simulink model "gm_uz_pmsm_model_9ph"  (R2021a)
settings: Solver=FixedStepAuto  StartTime=0.0  StopTime=.5  RelTol=1e-3
PreLoadFcn:
  | uz_pmsm_model_init_parameter
undefined symbols (not defined in the file or in its folder): friction_coefficient, inertia, k_i_d, k_p_d, k_p_q, L_d, L_o1, L_o2, L_q, L_x1, L_x2, L_y1, L_y2, L_zero, polepair, psi_pm, R_1, static_friction_torque
libraries: hdlmdlgenlib x220, hdlsllib x18, simulink x3, pid_lib x2
(part 1 of 4)
settings Model: Creator=ts  LastModifiedBy=valen
settings SolverCC: AlgebraicLoopSolver=TrustRegion  AutoInsertRateTranBlk=on
settings DataIOCC: LimitDataPoints=on  SaveOutput=off  SaveTime=off
settings OptimizationCC: BlockReduction=off  ConditionallyExecuteInputs=off  DefaultParameterBehavior=Inlined  LifeSpan=inf
settings DebuggingCC: AlgebraicLoopMsg=error  ArtificialAlgebraicLoopMsg=none  InheritedTsInSrcMsg=none  SingleTaskRateTransMsg=error  AllowSymbolicDim=off  StrictBusMsg=ErrorOnBusTreatedAsVector  SFUnexpectedBacktrackingDiag=warning  SFNoUnconditionalDefaultTransitionDiag=warning  SFExecutionAtInitializationDiag=none  SFMachineParentedDataDiag=warning  ArithmeticOperatorsInVariantConditions=warning
settings HardwareCC: ProdBitPerPointer=32  ProdBitPerSizeT=32  ProdBitPerPtrDiffT=32  ProdLargestAtomicFloat=None  ProdIntDivRoundTo=Undefined  ProdEndianess=Unspecified  ProdWordSize=32  ProdHWDeviceType=ASIC/FPGA->ASIC/FPGA  ProdEqTarget=off
settings SFSimCC: SimUseLocalCustomCode=off  CustomCodeUndefinedFunction=UseInterfaceOnly
settings RTWCC: RTWUseLocalCustomCode=off
settings CodeAppCC: StateflowObjectComments=on
settings GRTTargetCC: TargetLangStandard=C89/C90 (ANSI)
settings ConfigComp: CovScope=ReferencedModels  CovMetricSettings=dw  CovSaveCumulativeToWorkspaceVar=on  CovSaveSingleToWorkspaceVar=on  CovExternalEMLEnable=off  CovSFcnEnable=off

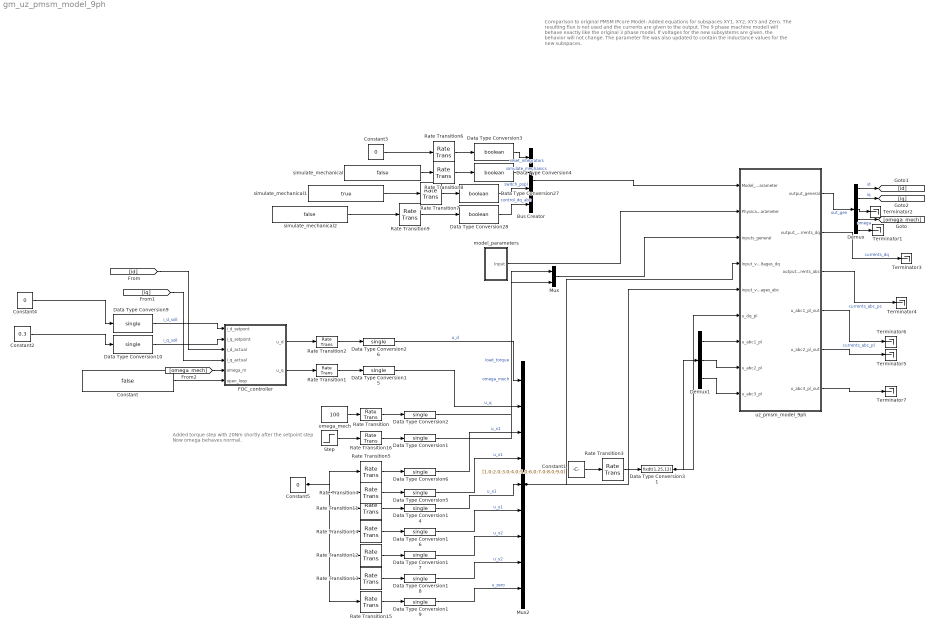
== system gm_uz_pmsm_model_9ph ==
  note: Comparison to original PMSM IPcore Model:
      | Added equations for subspaces XY1, XY2, XY3 and Zero. The resulting flux is not used and the currents are given to the output.
      | The 9 phase machine modell will behave exactly like the original 3 phase model. If voltages for the new subsystems are given, the behavior will not change.
      | The parameter file was also updated to contain the inductance values for the new subspaces.
  note: Added torque step with 20Nm shortly after the setpoint step
      | Now omega behaves normal.
  Bus Creator : BusCreator  Inputs=4
  Constant : Constant  Value=false
  Constant1 : Constant  Value=[1.0;2.0;3.0;4.0;5.0;6.0;7.0;8.0;9.0]
  Constant2 : Constant  Value=0.3
  Constant3 : Constant  Value=0
  Constant4 : Constant  Value=0
  Constant5 : Constant  Value=0
  Data Type Conversion{1..2,5..6,14..19,26} (11 alike) : DataTypeConversion  OutDataTypeStr=single  RndMeth=Nearest
  Data Type Conversion10 : DataTypeConversion  OutDataTypeStr=single
  Data Type Conversion{3..4,27..28} (4 alike) : DataTypeConversion  OutDataTypeStr=boolean
  Data Type Conversion31 : DataTypeConversion  OutDataTypeStr=fixdt(1,25,12)  RndMeth=Nearest
  Data Type Conversion9 : DataTypeConversion  OutDataTypeStr=single
  Demux : Demux  Outputs=5
  Demux1 : Demux  Outputs=3
  FOC_controller : Subsystem
  Mux : Mux  Inputs=2
  Mux2 : Mux  Inputs=9
  Rate Transition{,1..9,11..16} (16 alike) : RateTransition  OutPortSampleTime=ts
  Step : Step  Time=0.25  After=20  SampleTime=0
  Terminator{1..7} (7 alike) : Terminator
  model_parameters : Subsystem
  omega_mech : Constant  Value=100
  simulate_mechanical : Constant  Value=false
  simulate_mechanical1 : Constant  Value=true
  simulate_mechanical2 : Constant  Value=false
  uz_pmsm_model_9ph : Subsystem  TreatAsAtomicUnit=on
  wires:
  uz_pmsm_model_9ph/5(u_abc2_pl_out) -> Terminator5/1
  uz_pmsm_model_9ph/6(u_abc3_pl_out) -> Terminator7/1
  Demux1/3 -> uz_pmsm_model_9ph/9(u_abc3_pl)
  Demux1/2 -> uz_pmsm_model_9ph/8(u_abc2_pl)
  Demux1/1 -> uz_pmsm_model_9ph/7(u_abc1_pl)
  Rate Transition9/1 -> Data Type Conversion28/1
  Rate Transition7/1 -> Data Type Conversion27/1
  Data Type Conversion5/1 -> Mux2/4  "u_x1"
  Data Type Conversion6/1 -> Mux2/3  "u_x1"
  Rate Transition5/1 -> Data Type Conversion6/1
  Rate Transition4/1 -> Data Type Conversion5/1
  Data Type Conversion15/1 -> Mux2/2  "u_q"
  Data Type Conversion26/1 -> Mux2/1  "u_d"
  Demux/3 -> Terminator2/1
  Demux/5 -> Terminator1/1
  Constant2/1 -> Data Type Conversion10/1
  [id] -> FOC_controller/3(i_d_actual)
  [iq] -> FOC_controller/4(i_q_actual)
  Demux/2 -> [iq]  "iq"
  Demux/1 -> [id]  "id"
  Demux/4 -> [omega_mech]  "omega"
  [omega_mech] -> FOC_controller/5(omega_m)
  simulate_mechanical2/1 -> Rate Transition9/1
  simulate_mechanical1/1 -> Rate Transition7/1
  uz_pmsm_model_9ph/4(u_abc1_pl_out) -> Terminator6/1  "currents_abc_pl"
  Data Type Conversion31/1 -> uz_pmsm_model_9ph/6(u_dq_pl), Demux1/1
  Rate Transition3/1 -> Data Type Conversion31/1
  Constant1/1 -> Rate Transition3/1
  Data Type Conversion1/1 -> Mux/2  "load_torque"
  Data Type Conversion2/1 -> Mux/1  "omega_mech"
  Mux/1 -> uz_pmsm_model_9ph/3(inputs_general)
  Mux2/1 -> uz_pmsm_model_9ph/4(input_voltages_dq), uz_pmsm_model_9ph/5(input_voltages_abc)
  uz_pmsm_model_9ph/3(output_currents_abc) -> Terminator4/1  "currents_abc_ps"
  uz_pmsm_model_9ph/2(output_currents_dq) -> Terminator3/1  "currents_dq"
  Bus Creator/1 -> uz_pmsm_model_9ph/1(Model_Parameter)
  Data Type Conversion28/1 -> Bus Creator/4  "control_dq_abc"
  Data Type Conversion27/1 -> Bus Creator/3  "switch_pspl"
  Data Type Conversion3/1 -> Bus Creator/1  "reset_integrators"
  Data Type Conversion4/1 -> Bus Creator/2  "simulate_mechanics"
  model_parameters/1(Input) -> uz_pmsm_model_9ph/2(Physical_Parameter)
  Constant5/1 -> Rate Transition5/1, Rate Transition4/1, Rate Transition11/1, Rate Transition14/1, Rate Transition12/1, Rate Transition13/1, Rate Transition15/1
  Rate Transition15/1 -> Data Type Conversion19/1
  Data Type Conversion19/1 -> Mux2/9  "u_zero"
  Data Type Conversion18/1 -> Mux2/8  "u_y2"
  Data Type Conversion17/1 -> Mux2/7  "u_x2"
  Data Type Conversion16/1 -> Mux2/6  "u_y1"
  Rate Transition14/1 -> Data Type Conversion16/1
  Rate Transition12/1 -> Data Type Conversion17/1
  Rate Transition13/1 -> Data Type Conversion18/1
  Data Type Conversion14/1 -> Mux2/5  "u_x1"
  Rate Transition11/1 -> Data Type Conversion14/1
  Constant/1 -> FOC_controller/6(open_loop)
  omega_mech/1 -> Rate Transition/1
  FOC_controller/2(u_q) -> Rate Transition1/1
  FOC_controller/1(u_d) -> Rate Transition2/1
  Data Type Conversion10/1 -> FOC_controller/2(i_q_setpoint)  "i_q_soll"
  Data Type Conversion9/1 -> FOC_controller/1(i_d_setpont)  "i_d_soll"
  uz_pmsm_model_9ph/1(output_general) -> Demux/1  "out_gen"
  Constant4/1 -> Data Type Conversion9/1
  Rate Transition16/1 -> Data Type Conversion1/1
  Step/1 -> Rate Transition16/1
  simulate_mechanical/1 -> Rate Transition8/1
  Rate Transition8/1 -> Data Type Conversion4/1
  Constant3/1 -> Rate Transition6/1
  Rate Transition6/1 -> Data Type Conversion3/1
  Rate Transition2/1 -> Data Type Conversion26/1
  Rate Transition1/1 -> Data Type Conversion15/1
  Rate Transition/1 -> Data Type Conversion2/1

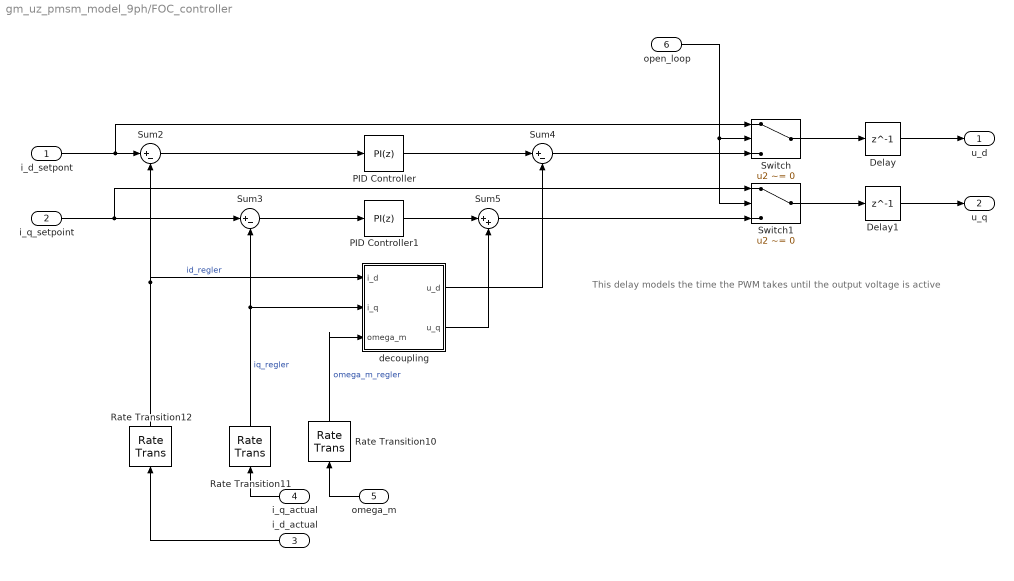
== system gm_uz_pmsm_model_9ph/FOC_controller ==
  note: This delay models the time the PWM takes until the output voltage is active
  i_d_setpont : Inport
  i_q_setpoint : Inport  Port=2
  i_d_actual : Inport  Port=3
  i_q_actual : Inport  Port=4
  omega_m : Inport  Port=5
  open_loop : Inport  Port=6
  Delay : Delay  DelayLength=1
  Delay1 : Delay  DelayLength=1
  PID Controller : pid_lib/PID Controller  Controller=PI  Form=Parallel  TimeDomain=Discrete-time  UseExternalTs=off  SampleTime=-1  IntegratorMethod=Forward Euler  FilterMethod=Forward Euler  ControllerParametersSource=internal  P=k_p_d  I=k_i_d  D=0  UseFilter=on  N=100  TunerSelectOption=Transfer Function Based (PID Tuner App)  InitialConditionSource=internal  InitialConditionForIntegrator=0  InitialConditionForFilter=0  DifferentiatorICPrevScaledInput=0  ExternalReset=none  TrackingMode=off  Kt=1  LimitOutput=off  SatLimitsSource=internal  UpperSaturationLimit=inf  LowerSaturationLimit=-inf  LinearizeAsGain=on  AntiWindupMode=none  Kb=1  POutMin=[]  POutMax=[]  IOutMin=[]  IOutMax=[]  DOutMin=[]  DOutMax=[]  NOutMin=[]  NOutMax=[]  SumOutMin=[]  SumOutMax=[]  SaturationOutMin=[]  SaturationOutMax=[]  PParamMin=[]  PParamMax=[]  IParamMin=[]  IParamMax=[]  DParamMin=[]  DParamMax=[]  NParamMin=[]  NParamMax=[]  KbParamMin=[]  KbParamMax=[]  KtParamMin=[]  KtParamMax=[]  KbOutMin=[]  KbOutMax=[]  KtOutMin=[]  KtOutMax=[]  IntegratorOutMin=[]  IntegratorOutMax=[]  FilterOutMin=[]  FilterOutMax=[]  SumI1OutMin=[]  SumI1OutMax=[]  SumI2OutMin=[]  SumI2OutMax=[]  SumI3OutMin=[]  SumI3OutMax=[]  SumI4OutMin=[]  SumI4OutMax=[]  SumDOutMin=[]  SumDOutMax=[]  DifferentiatorOutMin=[]  DifferentiatorOutMax=[]  FilterDiffOutCoefMin=[]  FilterDiffOutCoefMax=[]  ReciprocalOutMin=[]  ReciprocalOutMax=[]  SumDenOutMin=[]  SumDenOutMax=[]  SumNumOutMin=[]  SumNumOutMax=[]  DivideOutMin=[]  DivideOutMax=[]  UdiffTsProdOutMin=[]  UdiffTsProdOutMax=[]  NTsProdOutMin=[]  NTsProdOutMax=[]  UintegralTsProdOutMin=[]  UintegralTsProdOutMax=[]  UngainTsProdOutMin=[]  UngainTsProdOutMax=[]  IntegratorContinuousStateAttributes=''  IntegratorStateMustResolveToSignalObject=off  IntegratorRTWStateStorageClass=Auto  FilterContinuousStateAttributes=''  FilterStateMustResolveToSignalObject=off  FilterRTWStateStorageClass=Auto  ParallelPVariant=InternalParameters  IdealPVariant=Disabled  IVariant=InternalParameters  DVariant=Disabled  IntegratorVariant=Discrete  SatVariant=Disabled  AWVariant=Passthrough  PCopyVariant=Disabled  TRVariant=Disabled  FdbkBlocksVariant=Forward  IdealPFdbkVariant=Disabled  SatFdbkVariant=Disabled  DerivativeFilterVariant=Disabled  NVariant=Disabled  NCopyVariant=Disabled_SignalSpec  FilterICVariant=Disabled  IntegratorICVariant=InternalICs  ExternalResetVariant=Disabled  TRSumVariant=Passthrough  SumFdbkVariant=Disabled  SumVariant=Sum_PI  TsampFilterVariant=InternalTs  TsampNgainVariant=Passthrough  TsampIntegralVariant=Passthrough  ExternalSaturationOutDataTypeStr=Inherit: Same as second input
  PID Controller1 : pid_lib/PID Controller  Controller=PI  Form=Parallel  TimeDomain=Discrete-time  UseExternalTs=off  SampleTime=-1  IntegratorMethod=Forward Euler  FilterMethod=Forward Euler  ControllerParametersSource=internal  P=k_p_q  I=k_i_d  D=0  UseFilter=on  N=100  TunerSelectOption=Transfer Function Based (PID Tuner App)  InitialConditionSource=internal  InitialConditionForIntegrator=0  InitialConditionForFilter=0  DifferentiatorICPrevScaledInput=0  ExternalReset=none  TrackingMode=off  Kt=1  LimitOutput=off  SatLimitsSource=internal  UpperSaturationLimit=inf  LowerSaturationLimit=-inf  LinearizeAsGain=on  AntiWindupMode=none  Kb=1  POutMin=[]  POutMax=[]  IOutMin=[]  IOutMax=[]  DOutMin=[]  DOutMax=[]  NOutMin=[]  NOutMax=[]  SumOutMin=[]  SumOutMax=[]  SaturationOutMin=[]  SaturationOutMax=[]  PParamMin=[]  PParamMax=[]  IParamMin=[]  IParamMax=[]  DParamMin=[]  DParamMax=[]  NParamMin=[]  NParamMax=[]  KbParamMin=[]  KbParamMax=[]  KtParamMin=[]  KtParamMax=[]  KbOutMin=[]  KbOutMax=[]  KtOutMin=[]  KtOutMax=[]  IntegratorOutMin=[]  IntegratorOutMax=[]  FilterOutMin=[]  FilterOutMax=[]  SumI1OutMin=[]  SumI1OutMax=[]  SumI2OutMin=[]  SumI2OutMax=[]  SumI3OutMin=[]  SumI3OutMax=[]  SumI4OutMin=[]  SumI4OutMax=[]  SumDOutMin=[]  SumDOutMax=[]  DifferentiatorOutMin=[]  DifferentiatorOutMax=[]  FilterDiffOutCoefMin=[]  FilterDiffOutCoefMax=[]  ReciprocalOutMin=[]  ReciprocalOutMax=[]  SumDenOutMin=[]  SumDenOutMax=[]  SumNumOutMin=[]  SumNumOutMax=[]  DivideOutMin=[]  DivideOutMax=[]  UdiffTsProdOutMin=[]  UdiffTsProdOutMax=[]  NTsProdOutMin=[]  NTsProdOutMax=[]  UintegralTsProdOutMin=[]  UintegralTsProdOutMax=[]  UngainTsProdOutMin=[]  UngainTsProdOutMax=[]  IntegratorContinuousStateAttributes=''  IntegratorStateMustResolveToSignalObject=off  IntegratorRTWStateStorageClass=Auto  FilterContinuousStateAttributes=''  FilterStateMustResolveToSignalObject=off  FilterRTWStateStorageClass=Auto  ParallelPVariant=InternalParameters  IdealPVariant=Disabled  IVariant=InternalParameters  DVariant=Disabled  IntegratorVariant=Discrete  SatVariant=Disabled  AWVariant=Passthrough  PCopyVariant=Disabled  TRVariant=Disabled  FdbkBlocksVariant=Forward  IdealPFdbkVariant=Disabled  SatFdbkVariant=Disabled  DerivativeFilterVariant=Disabled  NVariant=Disabled  NCopyVariant=Disabled_SignalSpec  FilterICVariant=Disabled  IntegratorICVariant=InternalICs  ExternalResetVariant=Disabled  TRSumVariant=Passthrough  SumFdbkVariant=Disabled  SumVariant=Sum_PI  TsampFilterVariant=InternalTs  TsampNgainVariant=Passthrough  TsampIntegralVariant=Passthrough  ExternalSaturationOutDataTypeStr=Inherit: Same as second input
  Rate Transition10 : RateTransition  OutPortSampleTime=ts_regler
  Rate Transition11 : RateTransition  OutPortSampleTime=ts_regler
  Rate Transition12 : RateTransition  OutPortSampleTime=ts_regler
  Sum2 : Sum  Inputs=|+-
  Sum3 : Sum  Inputs=|+-
  Sum4 : Sum  Inputs=|+-
  Sum5 : Sum  Inputs=|++
  Switch : Switch  Criteria=u2 ~= 0
  Switch1 : Switch  Criteria=u2 ~= 0
  decoupling : Subsystem
  u_d : Outport
  u_q : Outport  Port=2
  wires:
  Delay1/1 -> u_q/1
  Delay/1 -> u_d/1
  Switch1/1 -> Delay1/1
  Switch/1 -> Delay/1
  decoupling/2(u_q) -> Sum5/2
  decoupling/1(u_d) -> Sum4/2
  Rate Transition10/1 -> decoupling/3(omega_m)  "omega_m_regler"
  open_loop/1 -> Switch/2, Switch1/2
  i_q_setpoint/1 -> Sum3/1, Switch1/1
  Rate Transition11/1 -> Sum3/2, decoupling/2(i_q)  "iq_regler"
  Rate Transition12/1 -> Sum2/2, decoupling/1(i_d)  "id_regler"
  i_q_actual/1 -> Rate Transition11/1
  Sum3/1 -> PID Controller1/1
  omega_m/1 -> Rate Transition10/1
  Sum5/1 -> Switch1/3
  Sum2/1 -> PID Controller/1
  i_d_setpont/1 -> Sum2/1, Switch/1
  i_d_actual/1 -> Rate Transition12/1
  Sum4/1 -> Switch/3
  PID Controller1/1 -> Sum5/1
  PID Controller/1 -> Sum4/1

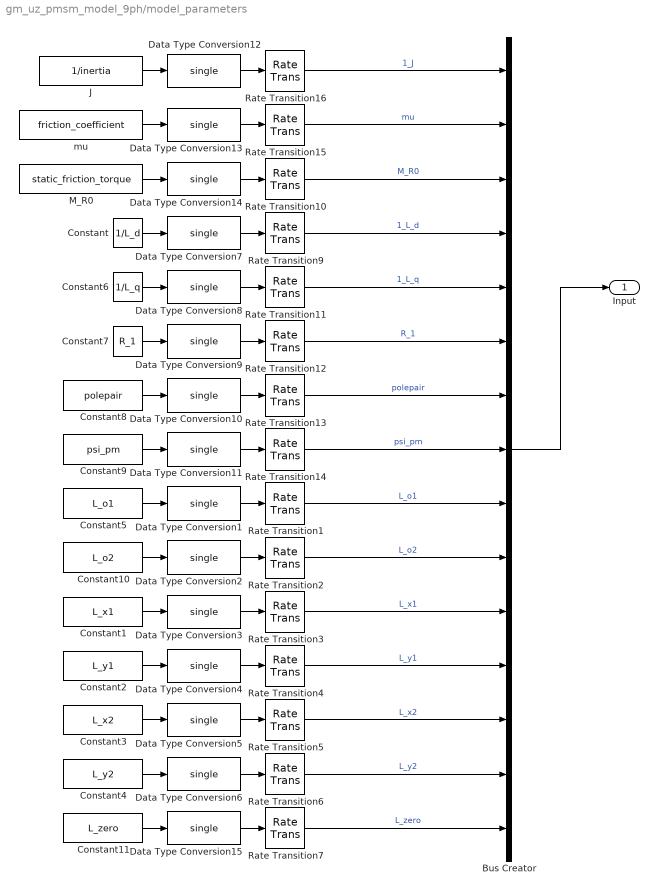
== system gm_uz_pmsm_model_9ph/model_parameters ==
  Bus Creator : BusCreator  Inputs=15
  Constant : Constant  Value=1/L_d
  Constant1 : Constant  Value=L_x1
  Constant10 : Constant  Value=L_o2
  Constant11 : Constant  Value=L_zero
  Constant2 : Constant  Value=L_y1
  Constant3 : Constant  Value=L_x2
  Constant4 : Constant  Value=L_y2
  Constant5 : Constant  Value=L_o1
  Constant6 : Constant  Value=1/L_q
  Constant7 : Constant  Value=R_1
  Constant8 : Constant  Value=polepair
  Constant9 : Constant  Value=psi_pm
  Data Type Conversion{1..15} (15 alike) : DataTypeConversion  OutDataTypeStr=single
  J : Constant  Value=1/inertia
  M_R0 : Constant  Value=static_friction_torque
  Rate Transition{1..7,9..16} (15 alike) : RateTransition  OutPortSampleTime=ts
  mu : Constant  Value=friction_coefficient
  Input : Outport
  wires:
  Constant10/1 -> Data Type Conversion2/1
  Constant5/1 -> Data Type Conversion1/1
  Constant1/1 -> Data Type Conversion3/1
  Constant2/1 -> Data Type Conversion4/1
  Constant3/1 -> Data Type Conversion5/1
  Constant4/1 -> Data Type Conversion6/1
  Rate Transition2/1 -> Bus Creator/10  "L_o2"
  Rate Transition3/1 -> Bus Creator/11  "L_x1"
  Rate Transition4/1 -> Bus Creator/12  "L_y1"
  Rate Transition5/1 -> Bus Creator/13  "L_x2"
  Rate Transition6/1 -> Bus Creator/14  "L_y2"
  Rate Transition7/1 -> Bus Creator/15  "L_zero"
  Rate Transition1/1 -> Bus Creator/9  "L_o1"
  Data Type Conversion15/1 -> Rate Transition7/1
  Constant11/1 -> Data Type Conversion15/1
  Data Type Conversion6/1 -> Rate Transition6/1
  Data Type Conversion5/1 -> Rate Transition5/1
  Data Type Conversion4/1 -> Rate Transition4/1
  Data Type Conversion3/1 -> Rate Transition3/1
  Data Type Conversion2/1 -> Rate Transition2/1
  Data Type Conversion1/1 -> Rate Transition1/1
  Constant/1 -> Data Type Conversion7/1
  Constant9/1 -> Data Type Conversion11/1
  Constant7/1 -> Data Type Conversion9/1
  Data Type Conversion13/1 -> Rate Transition15/1
  Rate Transition11/1 -> Bus Creator/5  "1_L_q"
  M_R0/1 -> Data Type Conversion14/1
  mu/1 -> Data Type Conversion13/1
  Data Type Conversion10/1 -> Rate Transition13/1
  Data Type Conversion8/1 -> Rate Transition11/1
  J/1 -> Data Type Conversion12/1
  Rate Transition9/1 -> Bus Creator/4  "1_L_d"
  Constant6/1 -> Data Type Conversion8/1
  Rate Transition15/1 -> Bus Creator/2  "mu"
  Data Type Conversion9/1 -> Rate Transition12/1
  Constant8/1 -> Data Type Conversion10/1
  Data Type Conversion11/1 -> Rate Transition14/1
  Bus Creator/1 -> Input/1
  Rate Transition13/1 -> Bus Creator/7  "polepair"
  Rate Transition16/1 -> Bus Creator/1  "1_J"
  Rate Transition12/1 -> Bus Creator/6  "R_1"
  Data Type Conversion14/1 -> Rate Transition10/1
  Rate Transition14/1 -> Bus Creator/8  "psi_pm"
  Rate Transition10/1 -> Bus Creator/3  "M_R0"
  Data Type Conversion7/1 -> Rate Transition9/1
  Data Type Conversion12/1 -> Rate Transition16/1
